simulink model "simulation"  (R2014a)
settings: Solver=ode45  StartTime=0.0  StopTime=10.0  RelTol=1e-3
settings Model: Creator=flp  LastModifiedBy=flp

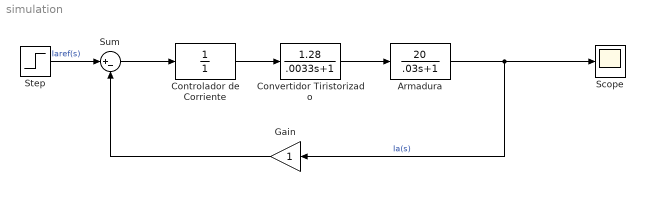
== system simulation ==
  Armadura : TransferFcn  Numerator=[20]  Denominator=[.03 1]
  Controlador de Corriente : TransferFcn  Denominator=[1]
  Convertidor Tiristorizado : TransferFcn  Numerator=[1.28]  Denominator=[.0033 1]
  Gain : Gain
  Scope : Scope
  Step : Step  SampleTime=0
  Sum : Sum  Inputs=|+-
  wires:
  Step/1 -> Sum/1  "Iaref(s)"
  Sum/1 -> Controlador de Corriente/1
  Controlador de Corriente/1 -> Convertidor Tiristorizado/1
  Convertidor Tiristorizado/1 -> Armadura/1
  Armadura/1 -> Gain/1, Scope/1  "Ia(s)"
  Gain/1 -> Sum/2
